simulink model "RLC_model"  (R2023a)
settings: Solver=VariableStepAuto  StartTime=0.0  StopTime=15  RelTol=1e-3
libraries: spspowerguiLib x1
settings Model: Creator=Ganesh Fashion  LastModifiedBy=Ganesh Fashion

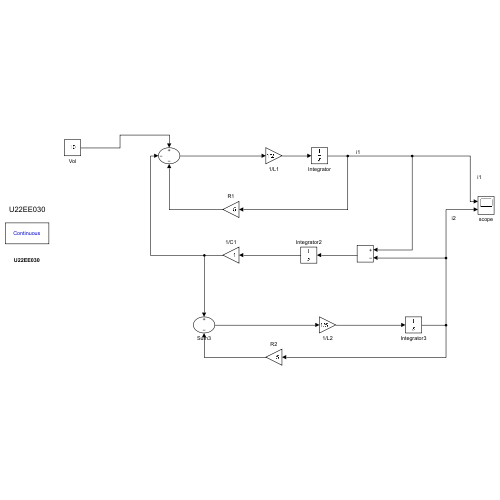
[thumbnail: Simulink's stored preview of the top-level diagram]
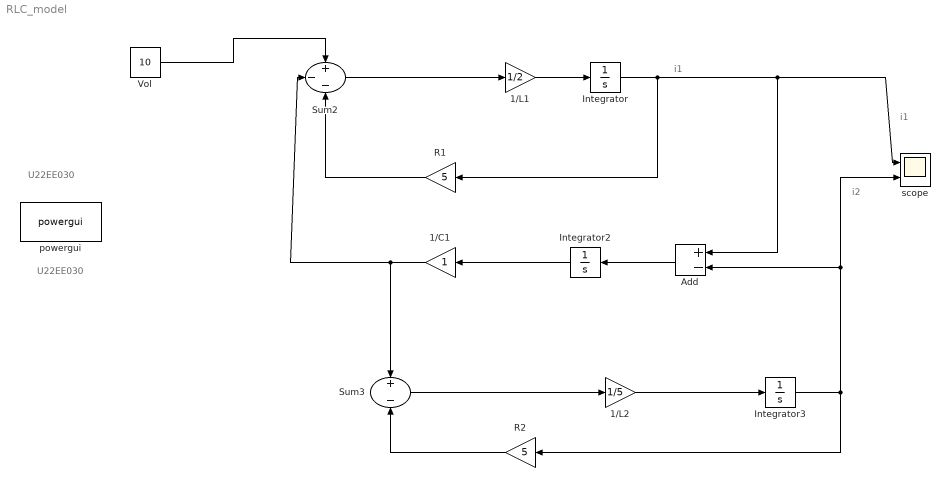
== system RLC_model ==
  note: U22EE030
  note: U22EE030
  note: i1
  note: i2
  note: i1
  1/C1 : Gain
  1/L1 : Gain  Gain=1/2
  1/L2 : Gain  Gain=1/5
  Add : Sum  Inputs=+-
  Integrator : Integrator
  Integrator2 : Integrator
  Integrator3 : Integrator
  R1 : Gain  Gain=5
  R2 : Gain  Gain=5
  Sum2 : Sum  Inputs=+--
  Sum3 : Sum  Inputs=+-
  Vol : Constant  Value=10
  powergui : spspowerguiLib/powergui  Priority=1  SimulationMode=Continuous  SampleTime=50e-6  frequency=60  Iterations=50  frequencyindice=60  Pbase=100e6  ErrMax=1e-4  UnitsV=kV  UnitsW=MW  buscounter=0  FunctionMessages=off  echomessages=off  EnableUseOfTLC=off  CurrentSourceSwitches=off  DisableSnubberDevices=off  DisableRonSwitches=off  DisableVfSwitches=off  DisplayEquations=off  AutomaticDiscreteSolvers=off  SolverType=Tustin/Backward Euler (TBE)  Interpol=off  ExternalGateDelay=off  methode=off  Ts=100  x0status=blocks  SPID=on  SwTol=0  HookPort=off  NonlinearTolerance=1e-4  nMaxIteration=100  ContinueOnMaxIteration=off  RestoreLinks=warning  ResistiveCurrentMeasurement=off  Frange=[0:2:500]  Ylog=off  Xlog=on  ShowGrid=off  save=off  variable=ZData  structure=0  ZoomFFT=off  StartTime=0.0  cycles=1  DisplayStyle=1  fundamental=60  FreqAxis=off  MaxFrequency=1000  frequencyindicesteady=1  RmsSteady=1  display=off
  scope : Scope  NumInputPorts=2
  wires:
  Vol/1 -> Sum2/1
  Sum2/1 -> 1/L1/1
  1/L1/1 -> Integrator/1
  R1/1 -> Sum2/3
  Integrator/1 -> R1/1, Add/1, scope/1
  1/C1/1 -> Sum2/2, Sum3/1
  Integrator2/1 -> 1/C1/1
  Add/1 -> Integrator2/1
  R2/1 -> Sum3/2
  Sum3/1 -> 1/L2/1
  1/L2/1 -> Integrator3/1
  Integrator3/1 -> R2/1, scope/2, Add/2
